simulink model "bh_lactose_model"  (R2018a)
settings: Solver=ode45  StartTime=0.0  StopTime=10.0  RelTol=1e-3
undefined symbols (not defined in the file): params_ode
libraries: simulink x3
settings Model: Creator=bhorton  LastModifiedBy=bhorton
settings DebuggingCC: SignalInfNanChecking=error  CheckMatrixSingularityMsg=error

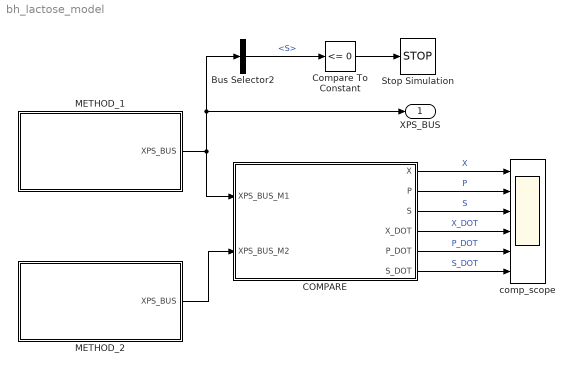
== system bh_lactose_model ==
  Bus Selector2 : BusSelector  OutputSignals=S
  COMPARE : Subsystem
  Compare To Constant : simulink/Logic and Bit Operations/Compare To Constant  relop=<=  const=0  OutDataTypeStr=boolean
  METHOD_1 : Subsystem
  METHOD_2 : Subsystem
  Stop Simulation : Stop
  comp_scope : Scope  NumInputPorts=6
  XPS_BUS : Outport
  wires:
  METHOD_1/1(XPS_BUS) -> Bus Selector2/1, XPS_BUS/1, COMPARE/1(XPS_BUS_M1)
  METHOD_2/1(XPS_BUS) -> COMPARE/2(XPS_BUS_M2)
  COMPARE/1(X) -> comp_scope/1  "X"
  COMPARE/2(P) -> comp_scope/2  "P"
  COMPARE/3(S) -> comp_scope/3  "S"
  COMPARE/4(X_DOT) -> comp_scope/4  "X_DOT"
  COMPARE/5(P_DOT) -> comp_scope/5  "P_DOT"
  COMPARE/6(S_DOT) -> comp_scope/6  "S_DOT"
  Bus Selector2/1 -> Compare To Constant/1  "<S>"
  Compare To Constant/1 -> Stop Simulation/1

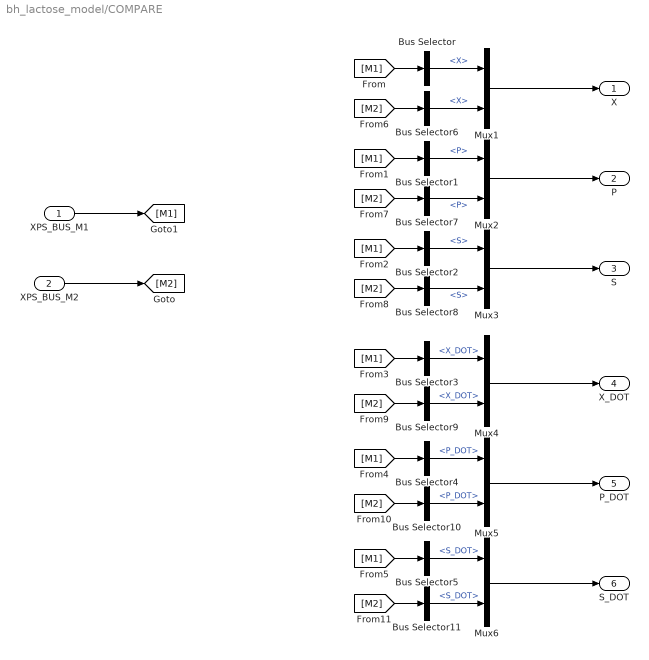
== system bh_lactose_model/COMPARE ==
  XPS_BUS_M1 : Inport
  XPS_BUS_M2 : Inport  Port=2
  Bus Selector : BusSelector  OutputSignals=X
  Bus Selector1 : BusSelector  OutputSignals=P
  Bus Selector10 : BusSelector  OutputSignals=P_DOT
  Bus Selector11 : BusSelector  OutputSignals=S_DOT
  Bus Selector2 : BusSelector  OutputSignals=S
  Bus Selector3 : BusSelector  OutputSignals=X_DOT
  Bus Selector4 : BusSelector  OutputSignals=P_DOT
  Bus Selector5 : BusSelector  OutputSignals=S_DOT
  Bus Selector6 : BusSelector  OutputSignals=X
  Bus Selector7 : BusSelector  OutputSignals=P
  Bus Selector8 : BusSelector  OutputSignals=S
  Bus Selector9 : BusSelector  OutputSignals=X_DOT
  Mux{1..6} (6 alike) : Mux  Inputs=2
  X : Outport
  P : Outport  Port=2
  S : Outport  Port=3
  X_DOT : Outport  Port=4
  P_DOT : Outport  Port=5
  S_DOT : Outport  Port=6
  wires:
  XPS_BUS_M1/1 -> [M1]
  XPS_BUS_M2/1 -> [M2]
  [M1] -> Bus Selector/1
  [M1] -> Bus Selector1/1
  [M1] -> Bus Selector2/1
  [M1] -> Bus Selector3/1
  [M1] -> Bus Selector4/1
  [M1] -> Bus Selector5/1
  [M2] -> Bus Selector6/1
  [M2] -> Bus Selector7/1
  [M2] -> Bus Selector8/1
  [M2] -> Bus Selector10/1
  [M2] -> Bus Selector11/1
  [M2] -> Bus Selector9/1
  Bus Selector6/1 -> Mux1/2  "<X>"
  Bus Selector/1 -> Mux1/1  "<X>"
  Bus Selector7/1 -> Mux2/2  "<P>"
  Bus Selector1/1 -> Mux2/1  "<P>"
  Bus Selector2/1 -> Mux3/1  "<S>"
  Bus Selector8/1 -> Mux3/2  "<S>"
  Bus Selector3/1 -> Mux4/1  "<X_DOT>"
  Bus Selector9/1 -> Mux4/2  "<X_DOT>"
  Bus Selector4/1 -> Mux5/1  "<P_DOT>"
  Bus Selector10/1 -> Mux5/2  "<P_DOT>"
  Bus Selector5/1 -> Mux6/1  "<S_DOT>"
  Bus Selector11/1 -> Mux6/2  "<S_DOT>"
  Mux6/1 -> S_DOT/1
  Mux5/1 -> P_DOT/1
  Mux4/1 -> X_DOT/1
  Mux1/1 -> X/1
  Mux2/1 -> P/1
  Mux3/1 -> S/1

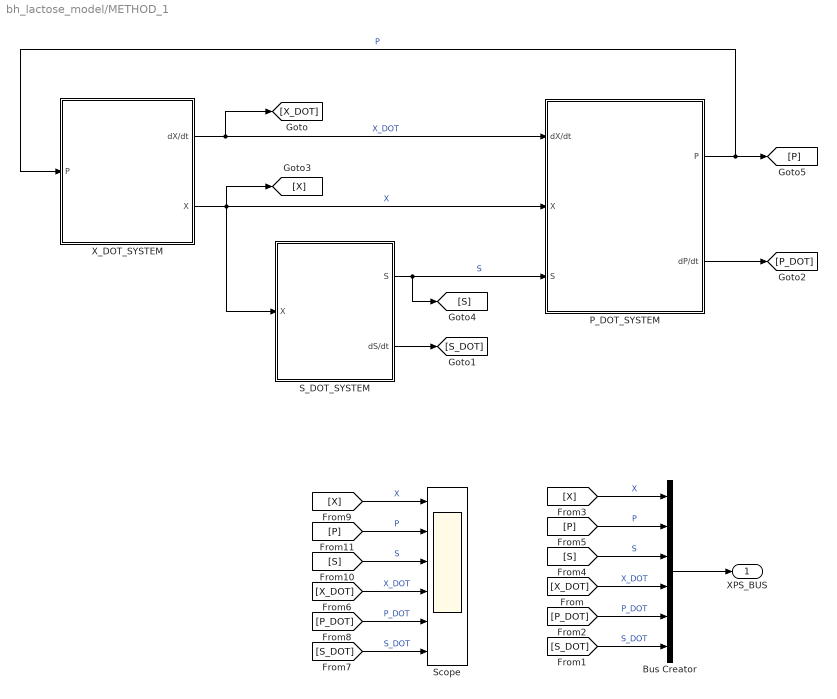
== system bh_lactose_model/METHOD_1 ==
  Bus Creator : BusCreator  Inputs=6
  P_DOT_SYSTEM : Subsystem
  S_DOT_SYSTEM : Subsystem
  Scope : Scope  NumInputPorts=6
  X_DOT_SYSTEM : Subsystem
  XPS_BUS : Outport
  wires:
  X_DOT_SYSTEM/1(dX/dt) -> P_DOT_SYSTEM/1(dX/dt), [X_DOT]  "X_DOT"
  P_DOT_SYSTEM/1(P) -> [P], X_DOT_SYSTEM/1(P)  "P"
  Bus Creator/1 -> XPS_BUS/1
  [S] -> Bus Creator/3  "S"
  X_DOT_SYSTEM/2(X) -> [X], S_DOT_SYSTEM/1(X), P_DOT_SYSTEM/2(X)  "X"
  P_DOT_SYSTEM/2(dP/dt) -> [P_DOT]
  [P] -> Scope/2  "P"
  [P] -> Bus Creator/2  "P"
  [P_DOT] -> Bus Creator/5  "P_DOT"
  [X_DOT] -> Bus Creator/4  "X_DOT"
  [X] -> Bus Creator/1  "X"
  [S_DOT] -> Bus Creator/6  "S_DOT"
  [X] -> Scope/1  "X"
  [S] -> Scope/3  "S"
  [P_DOT] -> Scope/5  "P_DOT"
  [X_DOT] -> Scope/4  "X_DOT"
  [S_DOT] -> Scope/6  "S_DOT"
  S_DOT_SYSTEM/1(S) -> P_DOT_SYSTEM/3(S), [S]  "S"
  S_DOT_SYSTEM/2(dS/dt) -> [S_DOT]

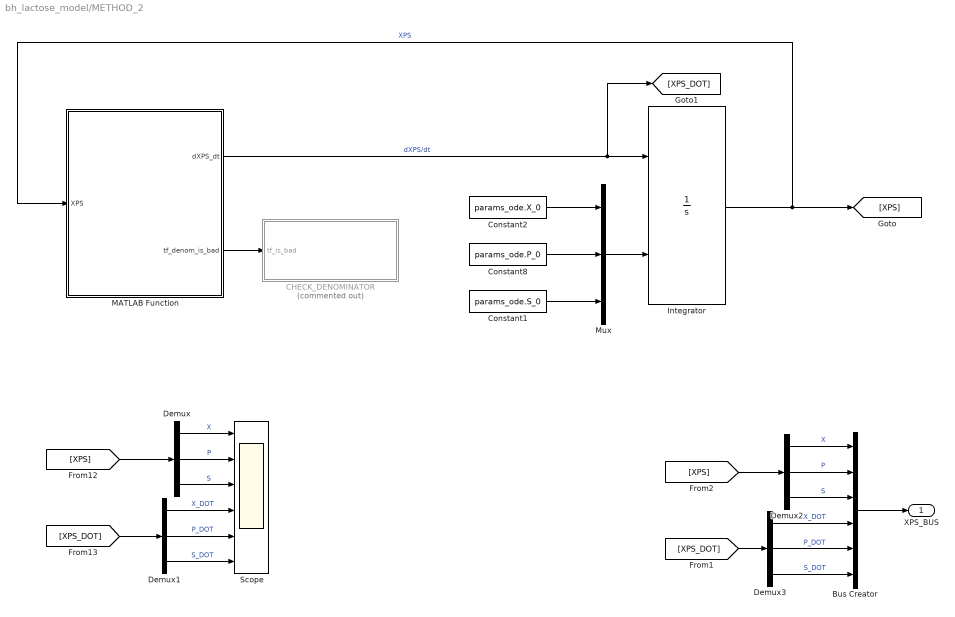
== system bh_lactose_model/METHOD_2 ==
  Bus Creator : BusCreator  Inputs=6
  CHECK_DENOMINATOR : Subsystem  Commented=on
  Constant1 : Constant  Value=params_ode.S_0
  Constant2 : Constant  Value=params_ode.X_0
  Constant8 : Constant  Value=params_ode.P_0
  Demux{,1..3} (4 alike) : Demux  Outputs=3
  Integrator : Integrator  InitialConditionSource=external
  MATLAB Function : MATLAB Function  TreatAsAtomicUnit=on
  Mux : Mux  Inputs=3
  Scope : Scope  NumInputPorts=6
  XPS_BUS : Outport
  wires:
  Bus Creator/1 -> XPS_BUS/1
  Demux2/3 -> Bus Creator/3  "S"
  Demux/2 -> Scope/2  "P"
  Demux2/2 -> Bus Creator/2  "P"
  Demux3/2 -> Bus Creator/5  "P_DOT"
  Demux3/1 -> Bus Creator/4  "X_DOT"
  Demux2/1 -> Bus Creator/1  "X"
  Demux3/3 -> Bus Creator/6  "S_DOT"
  Demux/1 -> Scope/1  "X"
  Demux/3 -> Scope/3  "S"
  Demux1/2 -> Scope/5  "P_DOT"
  Demux1/1 -> Scope/4  "X_DOT"
  Demux1/3 -> Scope/6  "S_DOT"
  MATLAB Function/1(dXPS_dt) -> Integrator/1, [XPS_DOT]  "dXPS/dt"
  Mux/1 -> Integrator/2
  Constant1/1 -> Mux/3
  Constant8/1 -> Mux/2
  Constant2/1 -> Mux/1
  Integrator/1 -> [XPS], MATLAB Function/1(XPS)  "XPS"
  [XPS] -> Demux/1
  [XPS_DOT] -> Demux1/1
  [XPS] -> Demux2/1
  [XPS_DOT] -> Demux3/1
  MATLAB Function/2(tf_denom_is_bad) -> CHECK_DENOMINATOR/1(tf_is_bad)

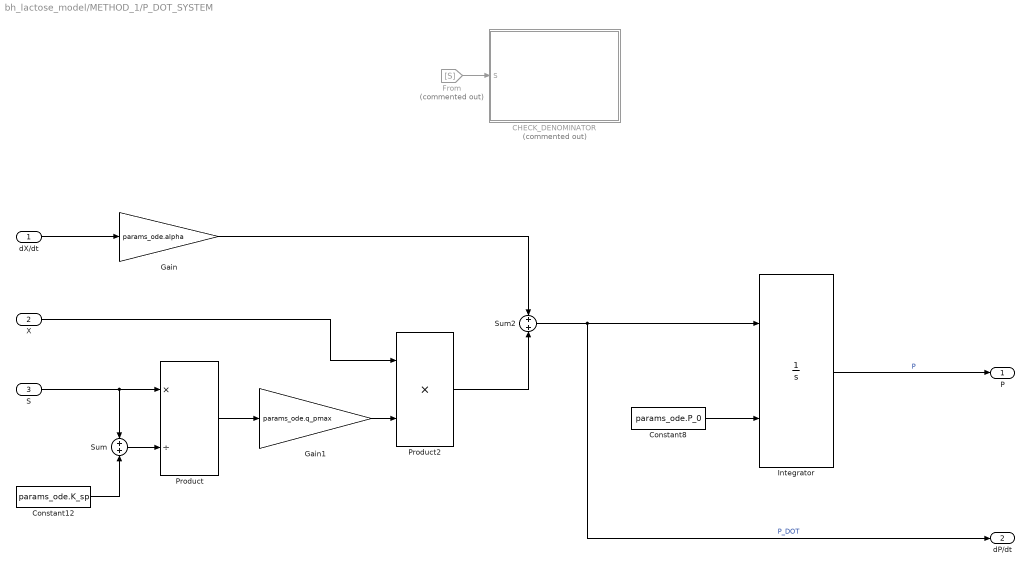
== system bh_lactose_model/METHOD_1/P_DOT_SYSTEM ==
  dX/dt : Inport
  X : Inport  Port=2
  S : Inport  Port=3
  CHECK_DENOMINATOR : Subsystem  Commented=on
  Constant12 : Constant  Value=params_ode.K_sp
  Constant8 : Constant  Value=params_ode.P_0
  From : From  Commented=on  GotoTag=S
  Gain : Gain  Gain=params_ode.alpha
  Gain1 : Gain  Gain=params_ode.q_pmax
  Integrator : Integrator  InitialConditionSource=external
  Product : Product  Inputs=*/
  Product2 : Product
  Sum : Sum  Inputs=+|+
  Sum2 : Sum  Inputs=+|+
  P : Outport
  dP/dt : Outport  Port=2
  wires:
  Constant8/1 -> Integrator/2
  Integrator/1 -> P/1  "P"
  Sum2/1 -> Integrator/1, dP/dt/1  "P_DOT"
  dX/dt/1 -> Gain/1
  S/1 -> Product/1, Sum/1
  Constant12/1 -> Sum/2
  Sum/1 -> Product/2
  Product/1 -> Gain1/1
  Gain1/1 -> Product2/2
  X/1 -> Product2/1
  Product2/1 -> Sum2/2
  Gain/1 -> Sum2/1
  From/1 -> CHECK_DENOMINATOR/1(S)

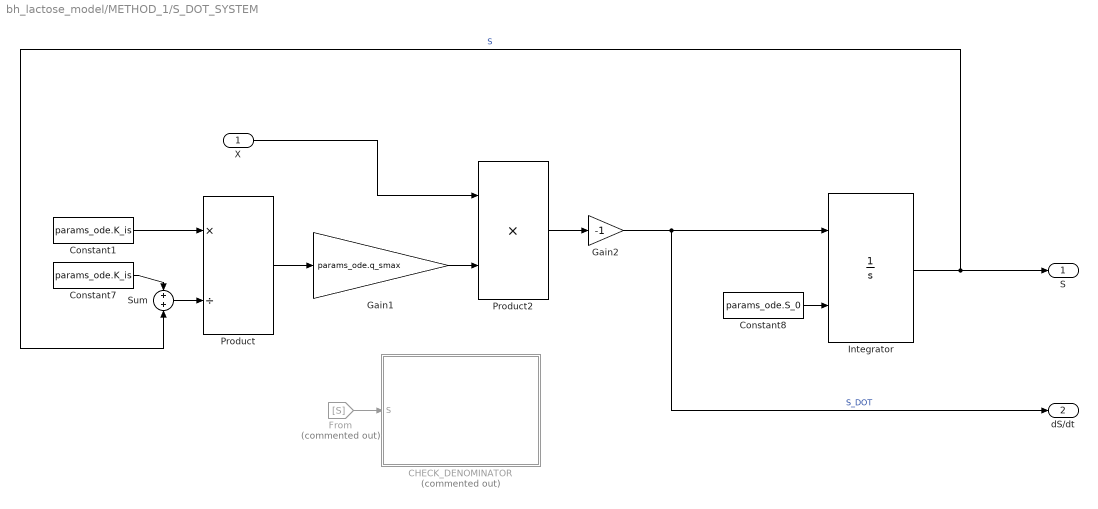
== system bh_lactose_model/METHOD_1/S_DOT_SYSTEM ==
  X : Inport
  CHECK_DENOMINATOR : Subsystem  Commented=on
  Constant1 : Constant  Value=params_ode.K_is
  Constant7 : Constant  Value=params_ode.K_is
  Constant8 : Constant  Value=params_ode.S_0
  From : From  Commented=on  GotoTag=S
  Gain1 : Gain  Gain=params_ode.q_smax
  Gain2 : Gain  Gain=-1
  Integrator : Integrator  InitialConditionSource=external
  Product : Product  Inputs=*/
  Product2 : Product
  Sum : Sum  Inputs=+|+
  S : Outport
  dS/dt : Outport  Port=2
  wires:
  Constant8/1 -> Integrator/2
  Integrator/1 -> Sum/2, S/1  "S"
  Sum/1 -> Product/2
  Product/1 -> Gain1/1
  Gain1/1 -> Product2/2
  X/1 -> Product2/1
  Constant7/1 -> Sum/1
  Constant1/1 -> Product/1
  Product2/1 -> Gain2/1
  Gain2/1 -> dS/dt/1, Integrator/1  "S_DOT"
  From/1 -> CHECK_DENOMINATOR/1(S)

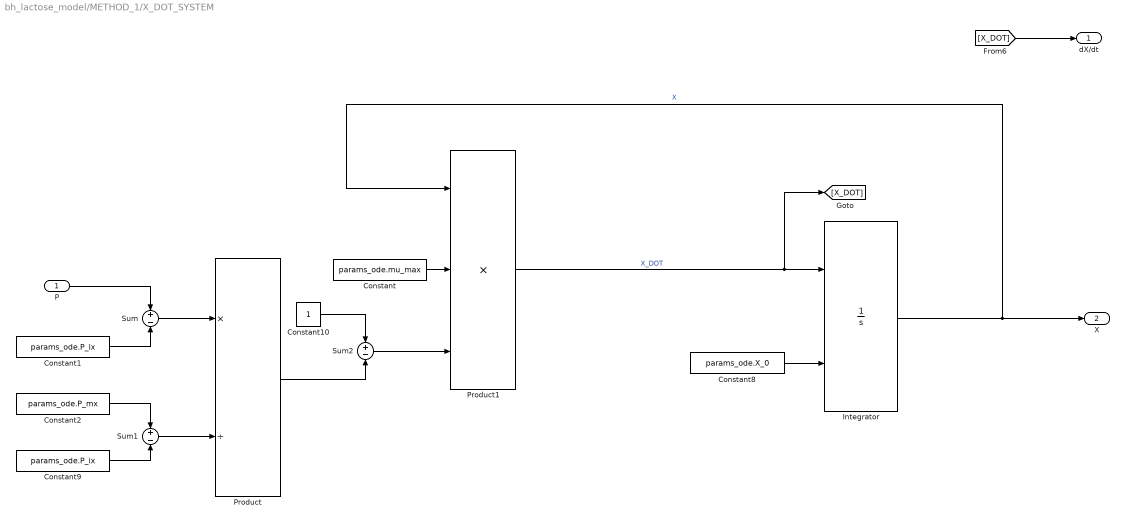
== system bh_lactose_model/METHOD_1/X_DOT_SYSTEM ==
  P : Inport
  Constant : Constant  Value=params_ode.mu_max
  Constant1 : Constant  Value=params_ode.P_ix
  Constant10 : Constant
  Constant2 : Constant  Value=params_ode.P_mx
  Constant8 : Constant  Value=params_ode.X_0
  Constant9 : Constant  Value=params_ode.P_ix
  Integrator : Integrator  InitialConditionSource=external
  Product : Product  Inputs=*/
  Product1 : Product  Inputs=3
  Sum : Sum  Inputs=+|-
  Sum1 : Sum  Inputs=+|-
  Sum2 : Sum  Inputs=+|-
  dX/dt : Outport
  X : Outport  Port=2
  wires:
  Constant8/1 -> Integrator/2
  Integrator/1 -> X/1, Product1/1  "X"
  P/1 -> Sum/1
  Constant1/1 -> Sum/2
  Sum/1 -> Product/1
  Constant9/1 -> Sum1/2
  Constant2/1 -> Sum1/1
  Sum1/1 -> Product/2
  Product/1 -> Sum2/2
  Constant10/1 -> Sum2/1
  Sum2/1 -> Product1/3
  Product1/1 -> [X_DOT], Integrator/1  "X_DOT"
  Constant/1 -> Product1/2
  [X_DOT] -> dX/dt/1

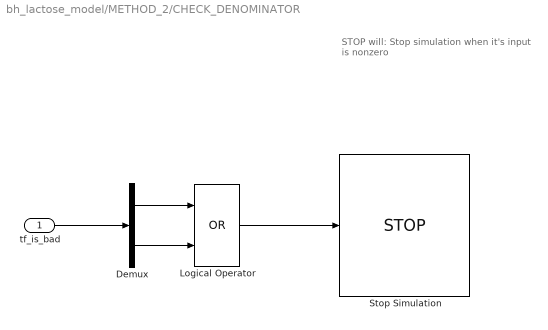
== system bh_lactose_model/METHOD_2/CHECK_DENOMINATOR ==
  note: STOP will:
      |
      | Stop simulation when
      | it's input is nonzero
  tf_is_bad : Inport
  Demux : Demux  Outputs=2
  Logical Operator : Logic  Operator=OR  AllPortsSameDT=off  OutDataTypeStr=boolean
  Stop Simulation : Stop
  wires:
  Logical Operator/1 -> Stop Simulation/1
  Demux/2 -> Logical Operator/2
  Demux/1 -> Logical Operator/1
  tf_is_bad/1 -> Demux/1

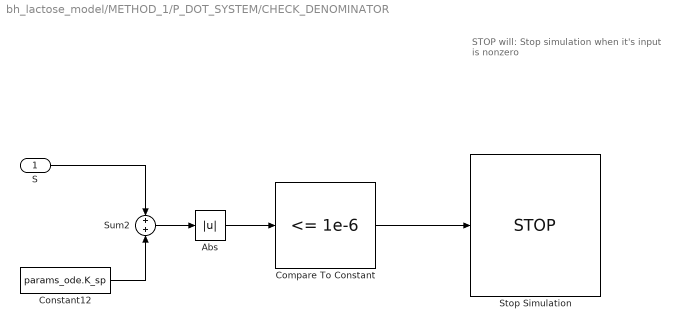
== system bh_lactose_model/METHOD_1/P_DOT_SYSTEM/CHECK_DENOMINATOR ==
  note: STOP will:
      |
      | Stop simulation when
      | it's input is nonzero
  S : Inport
  Abs : Abs
  Compare To Constant : simulink/Logic and Bit Operations/Compare To Constant  relop=<=  const=1e-6  OutDataTypeStr=boolean
  Constant12 : Constant  Value=params_ode.K_sp
  Stop Simulation : Stop
  Sum2 : Sum  Inputs=+|+
  wires:
  S/1 -> Sum2/1
  Constant12/1 -> Sum2/2
  Sum2/1 -> Abs/1
  Abs/1 -> Compare To Constant/1
  Compare To Constant/1 -> Stop Simulation/1

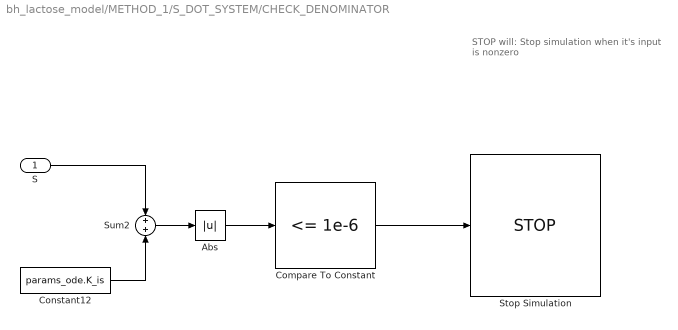
== system bh_lactose_model/METHOD_1/S_DOT_SYSTEM/CHECK_DENOMINATOR ==
  note: STOP will:
      |
      | Stop simulation when
      | it's input is nonzero
  S : Inport
  Abs : Abs
  Compare To Constant : simulink/Logic and Bit Operations/Compare To Constant  relop=<=  const=1e-6  OutDataTypeStr=boolean
  Constant12 : Constant  Value=params_ode.K_is
  Stop Simulation : Stop
  Sum2 : Sum  Inputs=+|+
  wires:
  S/1 -> Sum2/1
  Constant12/1 -> Sum2/2
  Sum2/1 -> Abs/1
  Abs/1 -> Compare To Constant/1
  Compare To Constant/1 -> Stop Simulation/1

== matlab function bh_lactose_model/METHOD_2/MATLAB Function ==
  data: XPS input; dXPS_dt output; params_ode parameter; tf_denom_is_bad output
function [dXPS_dt, tf_denom_is_bad] = my_odes(XPS, params_ode)

X      = XPS(1);
P      = XPS(2);
S      = XPS(3);

%% pull out the constant parameters
mu_max = params_ode.mu_max;
P_ix   = params_ode.P_ix;
P_mx   = params_ode.P_mx;
alpha  = params_ode.alpha;
q_pmax = params_ode.q_pmax;
K_sp   = params_ode.K_sp;
q_smax = params_ode.q_smax;
K_is   = params_ode.K_is;

%% check on the denominators for the P and S equations
% besides simply establishing that something BAD has happened
% we could of course use this understanding to do something sensible for
% the calculation of the derivatives(see NEXT section)
tf_denom_is_bad = [false, false];

if( abs(K_sp + S) <= 1e-6)
   tf_denom_is_bad(1) = true;
end

if( abs(K_is + S) <= 1e-6)
   tf_denom_is_bad(2) = true;
end

%% calculate derivatives.
dXdt = mu_max * X * ( 1 - (P - P_ix)/(P_mx - P_ix) );
dPdt = alpha*dXdt + q_pmax*X*S/(K_sp + S);
dSdt = -1*q_smax*X*K_is/(K_is + S);

%% take care of the OUTPUTS
dXPS_dt    = zeros(3,1);
dXPS_dt(1) = dXdt;
dXPS_dt(2) = dPdt;
dXPS_dt(3) = dSdt;

end % end of function
